simulink model "car_model"  (R2015b)
settings: Solver=VariableStepAuto  StartTime=0.0  StopTime=3.5  RelTol=1e-3
libraries: simulink x1
settings Model: Creator=Joran  LastModifiedBy=Joran

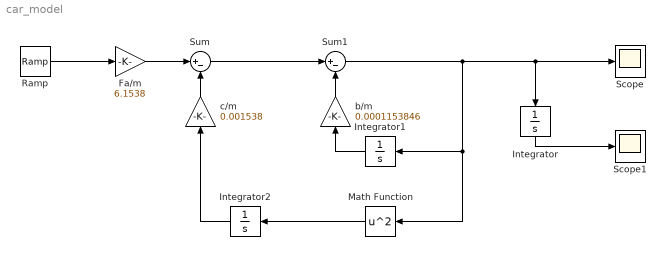
== system car_model ==
  Fa/m : Gain  Gain=6.1538
  Integrator : Integrator
  Integrator1 : Integrator
  Integrator2 : Integrator
  Math Function : Math  Operator=square  SaturateOnIntegerOverflow=on
  Ramp : simulink/Sources/Ramp  slope=1  start=0  X0=0
  Scope : Scope
  Scope1 : Scope
  Sum : Sum  Inputs=|+-
  Sum1 : Sum  Inputs=|+-
  b/m : Gain  Gain=0.0001153846
  c/m : Gain  Gain=0.001538
  wires:
  Fa/m/1 -> Sum/1
  Sum1/1 -> Math Function/1, Integrator1/1, Integrator/1, Scope/1
  Math Function/1 -> Integrator2/1
  Ramp/1 -> Fa/m/1
  c/m/1 -> Sum/2
  b/m/1 -> Sum1/2
  Sum/1 -> Sum1/1
  Integrator/1 -> Scope1/1
  Integrator1/1 -> b/m/1
  Integrator2/1 -> c/m/1
